simulink model "LongControl2"  (R2023a)
settings: Solver=VariableStepAuto  StartTime=0.0  StopTime=200  RelTol=1e-3
undefined symbols (not defined in the file or in its folder): accC, K, Kd, Kd1, Ki, Ki1, Kp, Kp1, N, N1, Ref, T, T1, tauh, torque, vstart
libraries: slpidlib x2, autolibshared x1
settings Model: Creator=brianlesko  LastModifiedBy=brianlesko
settings DataIOCC: ReturnWorkspaceOutputs=off

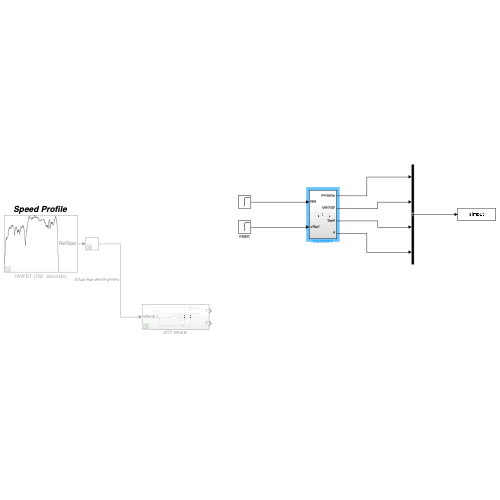
[thumbnail: Simulink's stored preview of the top-level diagram]
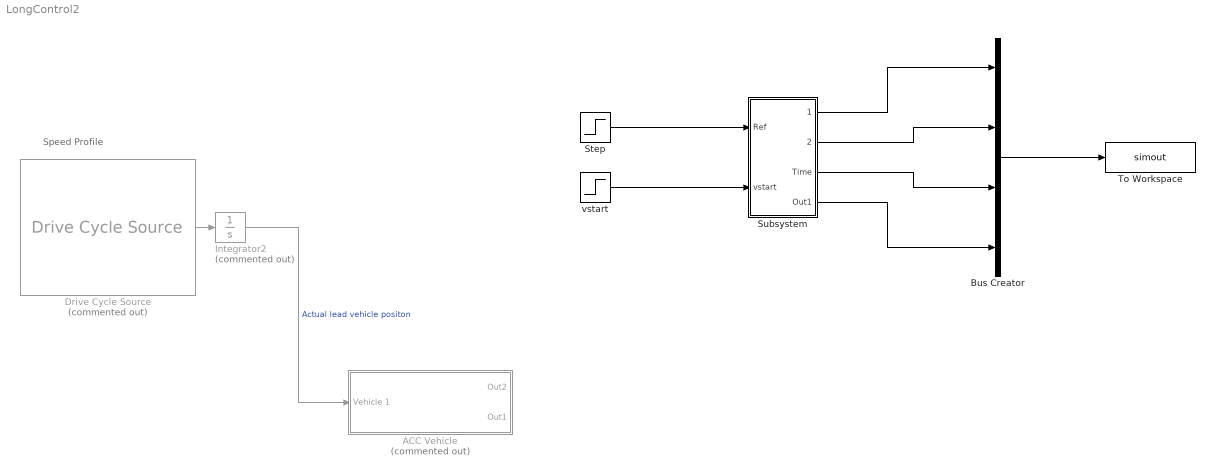
== system LongControl2 ==
  note: Speed Profile
  ACC Vehicle : Subsystem  Commented=on
  Bus Creator : BusCreator  Inputs=4
  Drive Cycle Source : autolibshared/Drive Cycle Source  Commented=on  cycleVar=HWFET  fileVar=cycleFTP75.mat  tfinal="765  seconds"  cycleRepeat=off  outAccPort=off  outGearPort=off  gearList=No gear data  t_wot1=5  xdot_woto=0  xdot_wot1=30  t_wot2=20  xdot_wot2=0  t_wotend=30  srcUnit=m/s  outUnit=m/s  srcAccUnit=m/s/s  outAccUnit=m/s^2  dt=0  aMode=2  faultOption=off  velBnd=2  velBndUnit=mph  inUnit=m/s  timeBnd=1  failOption=off  stopSim=off  maxFaultCnt=10  maxFaultTime=2  maxTotFaultTime=15  traceOption=off  dtTrace=1  traceWindow=10  lastDCname=HWFET  lastOutUnit=mph  lastDT=0  lastTB=1  lastSB=2  forceCalcBound=off
      settings: LibrarySourceBlock=vdynlib/Vehicle Scenarios/Drive Cycle and Maneuvers/Drive Cycle Source
  Integrator2 : Integrator  Commented=on
  Step : Step  Time=0  After=Ref  SampleTime=0
  Subsystem : Subsystem
  To Workspace : ToWorkspace  VariableName=simout  SampleTime=-1
  vstart : Step  Time=0  After=vstart  SampleTime=0
  wires:
  Integrator2/1 -> ACC Vehicle/1(Vehicle 1)  "Actual lead vehicle positon"
  Drive Cycle Source/1 -> Integrator2/1
  Subsystem/1(Position) -> Bus Creator/1
  Subsystem/2(Velocity) -> Bus Creator/2
  Subsystem/3(Time) -> Bus Creator/3
  Bus Creator/1 -> To Workspace/1
  Subsystem/4(Out1) -> Bus Creator/4
  Step/1 -> Subsystem/1(Ref)
  vstart/1 -> Subsystem/2(vstart)

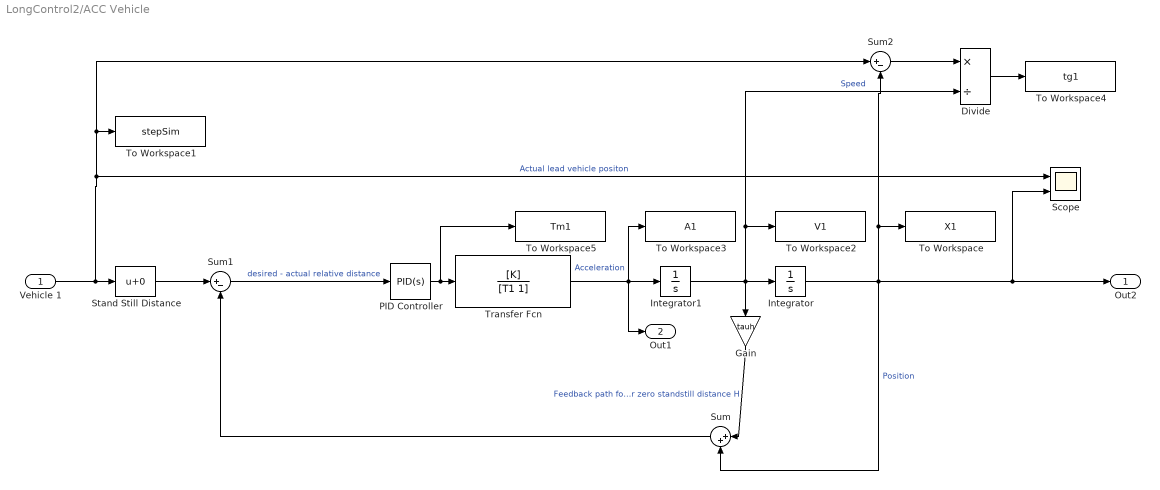
== system LongControl2/ACC Vehicle ==
  Vehicle 1 : Inport
  Divide : Product  Inputs=*/
  Gain : Gain  Gain=tauh
  Integrator : Integrator
  Integrator1 : Integrator
  PID Controller : slpidlib/PID Controller  Controller=PID  Form=Parallel  TimeDomain=Continuous-time  UseExternalTs=off  SampleTime=-1  IntegratorMethod=Forward Euler  FilterMethod=Forward Euler  ControllerParametersSource=internal  P=Kp1  I=Ki1  UseKiTs=off  D=Kd1  N=N1  UseFilter=on  TunerSelectOption=Transfer Function Based (PID Tuner App)  InitialConditionSource=internal  InitialConditionForIntegrator=0  InitialConditionForFilter=0  DifferentiatorICPrevScaledInput=0  ExternalReset=none  TrackingMode=off  Kt=1  LimitOutput=off  SatLimitsSource=internal  UpperSaturationLimit=inf  LowerSaturationLimit=-inf  LinearizeAsGain=on  AntiWindupMode=none  Kb=1  LimitIntegrator=off  UpperIntegratorSaturationLimit=inf  LowerIntegratorSaturationLimit=-inf  POutMin=[]  POutMax=[]  IOutMin=[]  IOutMax=[]  DOutMin=[]  DOutMax=[]  NOutMin=[]  NOutMax=[]  SumOutMin=[]  SumOutMax=[]  SaturationOutMin=[]  SaturationOutMax=[]  PParamMin=[]  PParamMax=[]  IParamMin=[]  IParamMax=[]  DParamMin=[]  DParamMax=[]  NParamMin=[]  NParamMax=[]  KbParamMin=[]  KbParamMax=[]  KtParamMin=[]  KtParamMax=[]  KbOutMin=[]  KbOutMax=[]  KtOutMin=[]  KtOutMax=[]  IntegratorOutMin=[]  IntegratorOutMax=[]  FilterOutMin=[]  FilterOutMax=[]  SumI1OutMin=[]  SumI1OutMax=[]  SumI2OutMin=[]  SumI2OutMax=[]  SumI3OutMin=[]  SumI3OutMax=[]  SumI4OutMin=[]  SumI4OutMax=[]  SumDOutMin=[]  SumDOutMax=[]  DifferentiatorOutMin=[]  DifferentiatorOutMax=[]  FilterDiffOutCoefMin=[]  FilterDiffOutCoefMax=[]  ReciprocalOutMin=[]  ReciprocalOutMax=[]  SumDenOutMin=[]  SumDenOutMax=[]  SumNumOutMin=[]  SumNumOutMax=[]  DivideOutMin=[]  DivideOutMax=[]  UdiffTsProdOutMin=[]  UdiffTsProdOutMax=[]  NTsProdOutMin=[]  NTsProdOutMax=[]  UintegralTsProdOutMin=[]  UintegralTsProdOutMax=[]  UngainTsProdOutMin=[]  UngainTsProdOutMax=[]  ClampingZeroOutDataTypeStr=Inherit: Inherit via back propagation  ClampingZeroOutMin=[]  ClampingZeroOutMax=[]  FilterDenConstantOutDataTypeStr=Inherit: Inherit via back propagation  FilterDenConstantOutMin=[]  FilterDenConstantOutMax=[]  PCopyOutDataTypeStr=Inherit: Inherit via back propagation  PCopyOutMin=[]  PCopyOutMax=[]  NCopyOutDataTypeStr=Inherit: Inherit via back propagation  NCopyOutMin=[]  NCopyOutMax=[]  IntegratorContinuousStateAttributes=''  IntegratorStateMustResolveToSignalObject=off  IntegratorRTWStateStorageClass=Auto  FilterContinuousStateAttributes=''  FilterStateMustResolveToSignalObject=off  FilterRTWStateStorageClass=Auto  ParallelPVariant=InternalParameters  IdealPVariant=Disabled  IVariant=InternalParameters  DVariant=InternalParameters  IntegratorVariant=Continuous  SatVariant=Disabled  AWVariant=Passthrough  PCopyVariant=Disabled  TRVariant=Disabled  FdbkBlocksVariant=Forward  IdealPFdbkVariant=Disabled  SatFdbkVariant=Disabled  DerivativeFilterVariant=ContFilter  NVariant=InternalParameters  NCopyVariant=Disabled  FilterICVariant=InternalICsFilter  IntegratorICVariant=InternalICs  ExternalResetVariant=Disabled  TRSumVariant=Passthrough  SumFdbkVariant=Disabled  SumVariant=Sum_PID  TsampFilterVariant=InternalTs  TsampNgainVariant=Passthrough  TsampIntegralVariant=Disabled_SignalSpec  ExternalSaturationOutDataTypeStr=Inherit: Same as second input
  Scope : Scope  NumInputPorts=2
  Stand Still Distance : Bias  SaturateOnIntegerOverflow=off
  Sum : Sum  Inputs=|++
  Sum1 : Sum  Inputs=|+-
  Sum2 : Sum  Inputs=|+-
  To Workspace : ToWorkspace  VariableName=X1  SampleTime=-1
      settings: Save2DSignal=2-D array (concatenate along first dimension)
  To Workspace1 : ToWorkspace  VariableName=stepSim  SampleTime=-1
  To Workspace2 : ToWorkspace  VariableName=V1  SampleTime=-1
  To Workspace3 : ToWorkspace  VariableName=A1  SampleTime=-1
  To Workspace4 : ToWorkspace  VariableName=tg1  SampleTime=-1
  To Workspace5 : ToWorkspace  VariableName=Tm1  SampleTime=-1
  Transfer Fcn : TransferFcn  Numerator=[K]  Denominator=[T1 1]
  Out2 : Outport
  Out1 : Outport  Port=2
  wires:
  Transfer Fcn/1 -> Out1/1, To Workspace3/1, Integrator1/1  "Acceleration"
  Gain/1 -> Sum/1  "Feedback path for zero standstill distance H"
  Stand Still Distance/1 -> Sum1/1
  Sum/1 -> Sum1/2
  Integrator/1 -> Out2/1, Scope/2, Sum/2, Sum2/2, To Workspace/1  "Position"
  PID Controller/1 -> To Workspace5/1, Transfer Fcn/1
  Sum1/1 -> PID Controller/1  "desired - actual relative distance"
  Integrator1/1 -> Integrator/1, Gain/1, Divide/2, To Workspace2/1  "Speed"
  Sum2/1 -> Divide/1
  Divide/1 -> To Workspace4/1
  Vehicle 1/1 -> Stand Still Distance/1, Scope/1, Sum2/1, To Workspace1/1  "Actual lead vehicle positon"

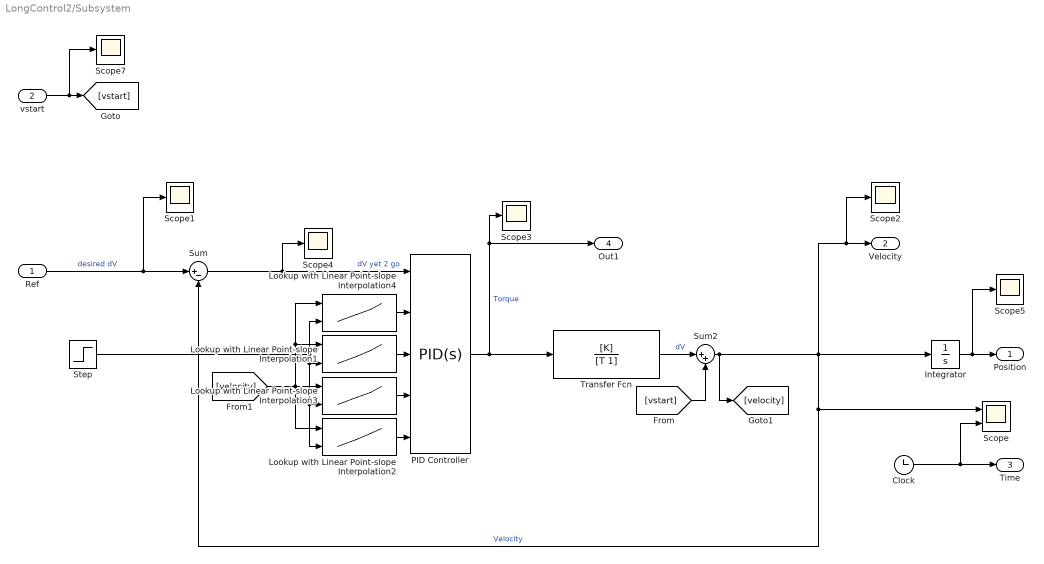
== system LongControl2/Subsystem ==
  Ref : Inport
  vstart : Inport  Port=2
  Clock : Clock
  Integrator : Integrator
  Lookup with Linear Point-slope Interpolation1 : Lookup_n-D  BreakpointsForDimension1=accC.Vs  BreakpointsForDimension2=accC.Tm_Tb  Table=accC.Ki  InternalRulePriority=Speed  RndMeth=Simplest
      settings: InputPortMap=u0,u1
  Lookup with Linear Point-slope Interpolation2 : Lookup_n-D  BreakpointsForDimension1=accC.Vs  BreakpointsForDimension2=accC.Tm_Tb  Table=accC.N  InternalRulePriority=Speed  RndMeth=Simplest
      settings: InputPortMap=u0,u1
  Lookup with Linear Point-slope Interpolation3 : Lookup_n-D  BreakpointsForDimension1=accC.Vs  BreakpointsForDimension2=accC.Tm_Tb  Table=accC.Kd  InternalRulePriority=Speed  RndMeth=Simplest
      settings: InputPortMap=u0,u1
  Lookup with Linear Point-slope Interpolation4 : Lookup_n-D  BreakpointsForDimension1=accC.Vs  BreakpointsForDimension2=accC.Tm_Tb  Table=accC.Kp  InternalRulePriority=Speed  RndMeth=Simplest
      settings: InputPortMap=u0,u1
  PID Controller : slpidlib/PID Controller  Controller=PID  Form=Parallel  TimeDomain=Continuous-time  UseExternalTs=off  SampleTime=-1  IntegratorMethod=Forward Euler  FilterMethod=Forward Euler  ControllerParametersSource=external  P=Kp  I=Ki  UseKiTs=off  D=Kd  N=N  UseFilter=on  TunerSelectOption=Transfer Function Based (PID Tuner App)  InitialConditionSource=internal  InitialConditionForIntegrator=0  InitialConditionForFilter=0  DifferentiatorICPrevScaledInput=0  ExternalReset=none  TrackingMode=off  Kt=1  LimitOutput=off  SatLimitsSource=internal  UpperSaturationLimit=inf  LowerSaturationLimit=-inf  LinearizeAsGain=on  AntiWindupMode=none  Kb=1  LimitIntegrator=off  UpperIntegratorSaturationLimit=inf  LowerIntegratorSaturationLimit=-inf  POutMin=[]  POutMax=[]  IOutMin=[]  IOutMax=[]  DOutMin=[]  DOutMax=[]  NOutMin=[]  NOutMax=[]  SumOutMin=[]  SumOutMax=[]  SaturationOutMin=[]  SaturationOutMax=[]  PParamMin=[]  PParamMax=[]  IParamMin=[]  IParamMax=[]  DParamMin=[]  DParamMax=[]  NParamMin=[]  NParamMax=[]  KbParamMin=[]  KbParamMax=[]  KtParamMin=[]  KtParamMax=[]  KbOutMin=[]  KbOutMax=[]  KtOutMin=[]  KtOutMax=[]  IntegratorOutMin=[]  IntegratorOutMax=[]  FilterOutMin=[]  FilterOutMax=[]  SumI1OutMin=[]  SumI1OutMax=[]  SumI2OutMin=[]  SumI2OutMax=[]  SumI3OutMin=[]  SumI3OutMax=[]  SumI4OutMin=[]  SumI4OutMax=[]  SumDOutMin=[]  SumDOutMax=[]  DifferentiatorOutMin=[]  DifferentiatorOutMax=[]  FilterDiffOutCoefMin=[]  FilterDiffOutCoefMax=[]  ReciprocalOutMin=[]  ReciprocalOutMax=[]  SumDenOutMin=[]  SumDenOutMax=[]  SumNumOutMin=[]  SumNumOutMax=[]  DivideOutMin=[]  DivideOutMax=[]  UdiffTsProdOutMin=[]  UdiffTsProdOutMax=[]  NTsProdOutMin=[]  NTsProdOutMax=[]  UintegralTsProdOutMin=[]  UintegralTsProdOutMax=[]  UngainTsProdOutMin=[]  UngainTsProdOutMax=[]  ClampingZeroOutDataTypeStr=Inherit: Inherit via back propagation  ClampingZeroOutMin=[]  ClampingZeroOutMax=[]  FilterDenConstantOutDataTypeStr=Inherit: Inherit via back propagation  FilterDenConstantOutMin=[]  FilterDenConstantOutMax=[]  PCopyOutDataTypeStr=Inherit: Inherit via back propagation  PCopyOutMin=[]  PCopyOutMax=[]  NCopyOutDataTypeStr=Inherit: Inherit via back propagation  NCopyOutMin=[]  NCopyOutMax=[]  IntegratorContinuousStateAttributes=''  IntegratorStateMustResolveToSignalObject=off  IntegratorRTWStateStorageClass=Auto  FilterContinuousStateAttributes=''  FilterStateMustResolveToSignalObject=off  FilterRTWStateStorageClass=Auto  ParallelPVariant=ExternalParameters  IdealPVariant=Disabled  IVariant=ExternalParameters  DVariant=ExternalParameters  IntegratorVariant=Continuous  SatVariant=Disabled  AWVariant=Passthrough  PCopyVariant=Disabled  TRVariant=Disabled  FdbkBlocksVariant=Forward  IdealPFdbkVariant=Disabled  SatFdbkVariant=Disabled  DerivativeFilterVariant=ContFilter  NVariant=ExternalParameters  NCopyVariant=Disabled  FilterICVariant=InternalICsFilter  IntegratorICVariant=InternalICs  ExternalResetVariant=Disabled  TRSumVariant=Passthrough  SumFdbkVariant=Disabled  SumVariant=Sum_PID  TsampFilterVariant=InternalTs  TsampNgainVariant=Passthrough  TsampIntegralVariant=Disabled_SignalSpec  ExternalSaturationOutDataTypeStr=Inherit: Same as second input
  Scope : Scope  NumInputPorts=2
  Scope{1..5,7} (6 alike) : Scope
  Step : Step  Time=0  After=torque  SampleTime=0
  Sum : Sum  Inputs=|+-
  Sum2 : Sum  Inputs=|++
  Transfer Fcn : TransferFcn  Numerator=[K]  Denominator=[T 1]
  Position : Outport
  Velocity : Outport  Port=2
  Time : Outport  Port=3
  Out1 : Outport  Port=4
  wires:
  Ref/1 -> Sum/1, Scope1/1  "desired dV"
  PID Controller/1 -> Scope3/1, Out1/1, Transfer Fcn/1  "Torque"
  Clock/1 -> Time/1, Scope/2
  Integrator/1 -> Scope5/1, Position/1
  Sum/1 -> Scope4/1, PID Controller/1  "dV yet 2 go"
  Sum2/1 -> [velocity], Sum/2, Scope/1, Integrator/1, Scope2/1, Velocity/1  "Velocity"
  [vstart] -> Sum2/2
  Transfer Fcn/1 -> Sum2/1  "dV"
  Lookup with Linear Point-slope Interpolation4/1 -> PID Controller/2
  Lookup with Linear Point-slope Interpolation1/1 -> PID Controller/3
  Lookup with Linear Point-slope Interpolation2/1 -> PID Controller/5
  Lookup with Linear Point-slope Interpolation3/1 -> PID Controller/4
  [velocity] -> Lookup with Linear Point-slope Interpolation3/1, Lookup with Linear Point-slope Interpolation2/1, Lookup with Linear Point-slope Interpolation1/1, Lookup with Linear Point-slope Interpolation4/1
  vstart/1 -> Scope7/1, [vstart]
  Step/1 -> Lookup with Linear Point-slope Interpolation4/2, Lookup with Linear Point-slope Interpolation2/2, Lookup with Linear Point-slope Interpolation3/2, Lookup with Linear Point-slope Interpolation1/2
